simulink model "DCmotor_modeling"  (R2015b)
settings: Solver=VariableStepAuto  StartTime=0.0  StopTime=5  RelTol=1e-3
values from neighbouring files (symbols this model uses):
  B = 0.1    [BLDCmotor_modeling_param.m]    (also in DCmotor_modeling_ss.m = [1/L; 0; 0])
  J = 0.1    [BLDCmotor_modeling_param.m]    (also in DCmotor_modeling_ss.m = 0.02)
  L = 0.1    [BLDCmotor_modeling_param.m]    (also in DCmotor_modeling_ss.m = 0.5)
  R = 0.02    [BLDCmotor_modeling_param.m]    (also in DCmotor_modeling_ss.m = 2)
undefined symbols (not defined in the file or in its folder): ke, kt
libraries: aerolibanimutils x1
settings Model: Creator=weberhsu  LastModifiedBy=root

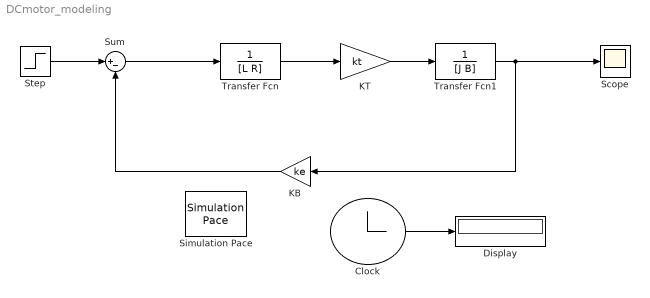
== system DCmotor_modeling ==
  Clock : Clock
  Display : Display
  KB : Gain  Gain=ke
  KT : Gain  Gain=kt
  Scope : Scope
  Simulation Pace : aerolibanimutils/Simulation Pace  SimulationPace=1  SleepMode=MATLAB Thread  OutputPaceError=off  SampleTime=1/30
  Step : Step  Time=0
  Sum : Sum  Inputs=|+-
  Transfer Fcn : TransferFcn  Denominator=[L R]
  Transfer Fcn1 : TransferFcn  Denominator=[J B]
  wires:
  Sum/1 -> Transfer Fcn/1
  Transfer Fcn/1 -> KT/1
  KT/1 -> Transfer Fcn1/1
  KB/1 -> Sum/2
  Step/1 -> Sum/1
  Transfer Fcn1/1 -> KB/1, Scope/1
  Clock/1 -> Display/1
